simulink model "pointing_group24"  (R2023b)
settings: Solver=FixedStepAuto  StartTime=0.0  StopTime=T  RelTol=1e-3
values from neighbouring files (symbols this model uses):
  a = 6939    [Air_Drag_script.m]    (also in main.m = 6939.063; main_group24.m = 6978)
  AccMagn = 0.5    [main_group24.m]
  AccSunSens = 0.125    [main_group24.m]
  ARW = deg2rad(0.10)    [main_group24.m]
  by = 0.1    [main_group24.m]
  bz = 0.1    [main_group24.m]
  c = 2.99792*10^8    (= 299792000)    [main.m]    (also in main_group24.m = 299792458)
  Cd = 2.2    [main_group24.m]
  e = 0    [Air_Drag_script.m]    (also in main.m = 0.001304; main_group24.m)
  G = [gn, gm, gvali, gsvi]    [main.m]    (also in main_group24.m)
  GyroSampleRate = 10    [main_group24.m]
  H = [hn, hm, hvali, hsvi]    [main.m]    (also in main_group24.m)
  H_0 = ((g1_0^2)+(g1_1^2)+(h1_1^2))^0.5    (= 2.98059244128e-05)    [main_group24.m]
  i = deg2rad(97.5307)    [Air_Drag_script.m]    (also in main.m; main_group24.m = deg2rad(98))
  I_tot = [Ix 0 0; 0 Iy 0; 0 0 Iz]    [data_mass.m]    (also in main_group24.m)
  invI_tot = inv(I_tot)    [data_mass.m]    (also in main_group24.m)
  Ix = J(1,1)    [Air_Drag_script.m]    (also in data_mass.m = 0.0755003333333; main.m = 0.057749855; main_group24.m = 0.0755003333333)
  Iy = J(2,2)    [Air_Drag_script.m]    (also in data_mass.m = 0.0755003333333; main.m = 0.04143542; main_group24.m = 0.0755003333333)
  Iz = J(3,3)    [Air_Drag_script.m]    (also in data_mass.m = 0.055; main.m = 0.024624309; main_group24.m = 0.055)
  k1 = 5e-2    (= 0.05)    [main_group24.m]
  k2 = 2.5e-2    (= 0.025)    [main_group24.m]
  m = [0.1; 0.1; 0.1]    [main.m]    (also in main_group24.m)
  MB = [4; 0.1; 0.1; 0.3]    [main.m]    (also in main_group24.m)
  MMnoise = 15e-9*[1; 1; 1]    [main_group24.m]
  MMSampleRate = 1    [main_group24.m]
  mu = 3.98600433e+5    (= 398600.433)    [main.m]    (also in main_group24.m)
  n = 0.0011    [Air_Drag_script.m]    (also in main.m = sqrt(mu/a^3); main_group24.m = sqrt(mu/a^3))
  n_E = 729.2e-07    (= 7.292e-05)    [main_group24.m]
  om_E = 0.000072921    (= 7.2921e-05)    [main_group24.m]
  P = Fe/c    (= 4.52980041279e-06)    [main_group24.m]
  q0 = [ 1 1 1 1 ]'    [Air_Drag_script.m]    (also in main_group24.m = [0 0 0 1]')
  R_e = 6378    [main.m]    (also in main_group24.m)
  rho_air = 1.65e-13    [Air_Drag_script.m]    (also in main_group24.m = 6.967e-13)
  rho_d_body = 0.1*2/3    (= 0.0666666666667)    [main_group24.m]
  rho_d_sp = 0.1*2/3    (= 0.0666666666667)    [main_group24.m]
  rho_s_body = 0.5    [main_group24.m]
  rho_s_sp = 0.1    [main_group24.m]
  RRW = deg2rad(0.3)    [main_group24.m]
  SP = [1; 0.3; 0.1; 0.01]    [main.m]    (also in main_group24.m = [0.25; 0.1; 0.3; 0.01])
undefined symbols (not defined in the file or in its folder): pan, s1, s2, s3, s4, s5, s6, thrust
libraries: vrlib x25, matrix_library x17, simulink_extras x8, sharedutil x3, simulink x1
(part 2 of 5)

== system pointing_group24/Sensors1/Magnetometer/Subsystem ==
  Constant : Constant
  Display : Display
  Gain : Gain  Gain=[1; -1; 1]
  Gain1 : Gain  Gain=[1; 1; -1]
  Gain2 : Gain  Gain=[-1; 1; 1]
  Matrix Concatenate : Concatenate  NumInputs=3  Mode=Multidimensional array  ConcatenateDimension=2
  Random Number : RandomNumber  Variance=deg2rad(0.1)^2  Seed=5  SampleTime=1/MMSampleRate
  Random Number1 : RandomNumber  Variance=deg2rad(0.1)^2  Seed=6  SampleTime=1/MMSampleRate
  Random Number2 : RandomNumber  Variance=deg2rad(0.1)^2  Seed=7  SampleTime=1/MMSampleRate
  Selector : Selector  InputPortWidth=4  IndexOptions=Index vector (dialog)  Indices=[1 4 3]  OutputSizes=1
  Selector1 : Selector  InputPortWidth=4  IndexOptions=Index vector (dialog)  Indices=[4 1 2]  OutputSizes=1
  Selector2 : Selector  InputPortWidth=4  IndexOptions=Index vector (dialog)  Indices=[3 2 1]  OutputSizes=1
  Vector Concatenate : Concatenate  NumInputs=4
  A_epsMM : Outport
  wires:
  Selector2/1 -> Gain2/1
  Selector/1 -> Gain/1
  Gain/1 -> Matrix Concatenate/1
  Random Number/1 -> Vector Concatenate/2
  Matrix Concatenate/1 -> Display/1, A_epsMM/1
  Selector1/1 -> Gain1/1
  Vector Concatenate/1 -> Selector2/1, Selector/1, Selector1/1
  Gain2/1 -> Matrix Concatenate/3
  Constant/1 -> Vector Concatenate/1
  Gain1/1 -> Matrix Concatenate/2
  Random Number2/1 -> Vector Concatenate/4
  Random Number1/1 -> Vector Concatenate/3

== system pointing_group24/Sensors1/Sun Sensor/Subsystem ==
  note: A31
  note: A33
  note: A32
  note: A23
  note: A22
  note: A21
  note: A13
  note: A12
  note: A11
  Cos : Trigonometry  Operator=cos
  Cos1 : Trigonometry  Operator=cos
  Cos2 : Trigonometry  Operator=cos
  Create 3x3 Matrix : sharedutil/Create 3x3 Matrix  aMode=aMode
  Gain1 : Gain  Gain=-1
  Gain3 : Gain  Gain=-1
  Gain4 : Gain
  Product{,1,3,5..6,8,10..11} (8 alike) : Product
  Product{2,4,7,9} (4 alike) : Product  Inputs=3
  Sin : Trigonometry
  Sin1 : Trigonometry
  Sin2 : Trigonometry
  Sum : Sum
  Sum1 : Sum  Inputs=-+
  Sum2 : Sum  Inputs=-+
  Sum3 : Sum
  phi : RandomNumber  Variance=(1/8*pi/180)^2  Seed=2  SampleTime=0.2
  psi : RandomNumber  Variance=(1/8*pi/180)^2  SampleTime=0.2
  th : RandomNumber  Variance=(1/8*pi/180)^2  Seed=1  SampleTime=0.2
  A_eps : Outport
  wires:
  psi/1 -> Cos/1, Sin/1
  th/1 -> Sin1/1, Cos1/1
  phi/1 -> Sin2/1, Cos2/1
  Product2/1 -> Sum/1
  Product1/1 -> Sum/2
  Product3/1 -> Sum1/2
  Product4/1 -> Sum1/1
  Product7/1 -> Sum2/1
  Product6/1 -> Sum2/2
  Product9/1 -> Sum3/1
  Product8/1 -> Sum3/2
  Gain4/1 -> Create 3x3 Matrix/7  "A31"
  Product/1 -> Create 3x3 Matrix/1  "A11"
  Sum/1 -> Create 3x3 Matrix/2  "A12"
  Sum1/1 -> Create 3x3 Matrix/3  "A13"
  Product5/1 -> Gain1/1
  Sum2/1 -> Create 3x3 Matrix/5  "A22"
  Sum3/1 -> Create 3x3 Matrix/6  "A23"
  Product10/1 -> Gain3/1
  Product11/1 -> Create 3x3 Matrix/9  "A33"
  Gain1/1 -> Create 3x3 Matrix/4  "A21"
  Gain3/1 -> Create 3x3 Matrix/8  "A32"
  Cos/1 -> Product8/1, Product6/1, Product4/1, Product2/1, Product/1  "cos(psi)"
  Cos1/1 -> Product/2, Product11/1, Product10/1, Product5/2  "cos(th)"
  Sin1/1 -> Gain4/1, Product9/2, Product7/2, Product2/2, Product4/2  "sin(th)"
  Sin2/1 -> Product7/3, Product3/2, Product2/3, Product8/2, Product10/2  "sin(phi)"
  Sin/1 -> Product3/1, Product5/1, Product7/1, Product9/1, Product1/1  "sin(psi)"
  Cos2/1 -> Product6/2, Product4/3, Product1/2, Product9/3, Product11/2  "cos(phi)"
  Create 3x3 Matrix/1 -> A_eps/1  "A_eps"

== system pointing_group24/Attitude Control/Ideal controller/Subsystem2/Subsystem ==
  A11 : Inport
  A12 : Inport  Port=2
  A13 : Inport  Port=3
  A21 : Inport  Port=4
  A22 : Inport  Port=5
  A23 : Inport  Port=6
  A31 : Inport  Port=7
  A32 : Inport  Port=8
  A33 : Inport  Port=9
  Matrix Concatenate : Concatenate  NumInputs=3  Mode=Multidimensional array  ConcatenateDimension=2
  Mux : Mux  Inputs=3
  Mux1 : Mux  Inputs=3
  Mux2 : Mux  Inputs=3
  A_BN_312 : Outport
  wires:
  A31/1 -> Mux/3
  A13/1 -> Mux2/1
  Matrix Concatenate/1 -> A_BN_312/1
  Mux1/1 -> Matrix Concatenate/2
  A21/1 -> Mux/2
  A11/1 -> Mux/1
  A32/1 -> Mux1/3
  A12/1 -> Mux1/1
  Mux/1 -> Matrix Concatenate/1
  A33/1 -> Mux2/3
  A22/1 -> Mux1/2
  A23/1 -> Mux2/2
  Mux2/1 -> Matrix Concatenate/3

== system pointing_group24/Desturbances/External Torques/Air Drag/Subsystem ==
  v_rel_N^2 : Inport
  v_rel_B : Inport  Port=2
  Constant : Constant  Value=-0.5
  Constant1 : Constant  Value=s1.n
  Constant2 : Constant  Value=s1.r
  Constant3 : Constant  Value=s1.A
  Cross Product2 : vrlib/Utilities/Cross Product
  Dot Product1 : DotProduct  OutDataTypeStr=Inherit: Inherit via internal rule
  Gain : Gain  Gain=rho_air
  Gain1 : Gain  Gain=0
  Gain2 : Gain  Gain=Cd
  Product : Product  Inputs=5
  Switch1 : Switch  Criteria=u2 > Threshold  SaturateOnIntegerOverflow=off  InputSameDT=off
  Pan1 : Outport
  wires:
  Constant2/1 -> Cross Product2/1
  Gain1/1 -> Switch1/3
  Dot Product1/1 -> Gain1/1, Switch1/2, Switch1/1
  Constant3/1 -> Product/2
  Product/1 -> Cross Product2/2
  Switch1/1 -> Product/5
  v_rel_B/1 -> Dot Product1/1, Product/4
  Gain/1 -> Gain2/1
  Constant/1 -> Gain/1
  Cross Product2/1 -> Pan1/1
  Constant1/1 -> Dot Product1/2
  Gain2/1 -> Product/1
  v_rel_N^2/1 -> Product/3

== system pointing_group24/Desturbances/External Torques/Air Drag/Subsystem1 ==
  v_rel_N^2 : Inport
  v_rel_B : Inport  Port=2
  Constant : Constant  Value=-0.5
  Constant1 : Constant  Value=s2.n
  Constant2 : Constant  Value=s2.r
  Constant3 : Constant  Value=s2.A
  Cross Product2 : vrlib/Utilities/Cross Product
  Dot Product1 : DotProduct  OutDataTypeStr=Inherit: Inherit via internal rule
  Gain : Gain  Gain=rho_air
  Gain1 : Gain  Gain=0
  Gain2 : Gain  Gain=Cd
  Product : Product  Inputs=5
  Switch1 : Switch  Criteria=u2 > Threshold  SaturateOnIntegerOverflow=off  InputSameDT=off
  Pan2 : Outport
  wires:
  Constant1/1 -> Dot Product1/2
  Cross Product2/1 -> Pan2/1
  Constant/1 -> Gain/1
  Gain/1 -> Gain2/1
  Gain2/1 -> Product/1
  v_rel_B/1 -> Product/4, Dot Product1/1
  Switch1/1 -> Product/5
  Product/1 -> Cross Product2/2
  Constant3/1 -> Product/2
  Dot Product1/1 -> Switch1/1, Switch1/2, Gain1/1
  Gain1/1 -> Switch1/3
  Constant2/1 -> Cross Product2/1
  v_rel_N^2/1 -> Product/3

== system pointing_group24/Desturbances/External Torques/Air Drag/Subsystem2 ==
  v_rel_N^2 : Inport
  v_rel_B : Inport  Port=2
  Constant : Constant  Value=-0.5
  Constant1 : Constant  Value=s3.n
  Constant2 : Constant  Value=s3.r
  Constant3 : Constant  Value=s3.A
  Cross Product2 : vrlib/Utilities/Cross Product
  Dot Product1 : DotProduct  OutDataTypeStr=Inherit: Inherit via internal rule
  Gain : Gain  Gain=rho_air
  Gain1 : Gain  Gain=0
  Gain2 : Gain  Gain=Cd
  Product : Product  Inputs=5
  Switch1 : Switch  Criteria=u2 > Threshold  SaturateOnIntegerOverflow=off  InputSameDT=off
  Pan3 : Outport
  wires:
  Constant2/1 -> Cross Product2/1
  Gain1/1 -> Switch1/3
  Dot Product1/1 -> Gain1/1, Switch1/2, Switch1/1
  Constant3/1 -> Product/2
  Product/1 -> Cross Product2/2
  Switch1/1 -> Product/5
  v_rel_B/1 -> Dot Product1/1, Product/4
  Gain2/1 -> Product/1
  Gain/1 -> Gain2/1
  Constant/1 -> Gain/1
  Cross Product2/1 -> Pan3/1
  Constant1/1 -> Dot Product1/2
  v_rel_N^2/1 -> Product/3

== system pointing_group24/Desturbances/External Torques/Air Drag/Subsystem3 ==
  v_rel_N^2 : Inport
  v_rel_B : Inport  Port=2
  Constant : Constant  Value=-0.5
  Constant1 : Constant  Value=s4.n
  Constant2 : Constant  Value=s4.r
  Constant3 : Constant  Value=s4.A
  Cross Product2 : vrlib/Utilities/Cross Product
  Dot Product1 : DotProduct  OutDataTypeStr=Inherit: Inherit via internal rule
  Gain : Gain  Gain=rho_air
  Gain1 : Gain  Gain=0
  Gain2 : Gain  Gain=Cd
  Product : Product  Inputs=5
  Switch1 : Switch  Criteria=u2 > Threshold  SaturateOnIntegerOverflow=off  InputSameDT=off
  Pan4 : Outport
  wires:
  Constant1/1 -> Dot Product1/2
  Cross Product2/1 -> Pan4/1
  Constant/1 -> Gain/1
  Gain/1 -> Gain2/1
  Gain2/1 -> Product/1
  v_rel_B/1 -> Product/4, Dot Product1/1
  Switch1/1 -> Product/5
  Product/1 -> Cross Product2/2
  Constant3/1 -> Product/2
  Dot Product1/1 -> Switch1/1, Switch1/2, Gain1/1
  Gain1/1 -> Switch1/3
  Constant2/1 -> Cross Product2/1
  v_rel_N^2/1 -> Product/3

== system pointing_group24/Desturbances/External Torques/Air Drag/Subsystem4 ==
  v_rel_N^2 : Inport
  v_rel_B : Inport  Port=2
  Constant : Constant  Value=-0.5
  Constant1 : Constant  Value=s5.n
  Constant2 : Constant  Value=s5.r
  Constant3 : Constant  Value=s5.A
  Cross Product2 : vrlib/Utilities/Cross Product
  Dot Product1 : DotProduct  OutDataTypeStr=Inherit: Inherit via internal rule
  Gain : Gain  Gain=rho_air
  Gain1 : Gain  Gain=0
  Gain2 : Gain  Gain=Cd
  Product : Product  Inputs=5
  Switch1 : Switch  Criteria=u2 > Threshold  SaturateOnIntegerOverflow=off  InputSameDT=off
  Pan5 : Outport
  wires:
  Constant2/1 -> Cross Product2/1
  Gain1/1 -> Switch1/3
  Dot Product1/1 -> Gain1/1, Switch1/2, Switch1/1
  Constant3/1 -> Product/2
  Product/1 -> Cross Product2/2
  Switch1/1 -> Product/5
  v_rel_B/1 -> Dot Product1/1, Product/4
  Gain2/1 -> Product/1
  Gain/1 -> Gain2/1
  Constant/1 -> Gain/1
  Cross Product2/1 -> Pan5/1
  Constant1/1 -> Dot Product1/2
  v_rel_N^2/1 -> Product/3

== system pointing_group24/Desturbances/External Torques/Air Drag/Subsystem5 ==
  v_rel_N^2 : Inport
  v_rel_B : Inport  Port=2
  Constant : Constant  Value=-0.5
  Constant1 : Constant  Value=s6.n
  Constant2 : Constant  Value=s6.r
  Constant3 : Constant  Value=s6.A
  Cross Product2 : vrlib/Utilities/Cross Product
  Dot Product1 : DotProduct  OutDataTypeStr=Inherit: Inherit via internal rule
  Gain : Gain  Gain=rho_air
  Gain1 : Gain  Gain=0
  Gain2 : Gain  Gain=Cd
  Product : Product  Inputs=5
  Switch1 : Switch  Criteria=u2 > Threshold  SaturateOnIntegerOverflow=off  InputSameDT=off
  Pan6 : Outport
  wires:
  Constant2/1 -> Cross Product2/1
  Gain1/1 -> Switch1/3
  Dot Product1/1 -> Gain1/1, Switch1/2, Switch1/1
  Constant3/1 -> Product/2
  Product/1 -> Cross Product2/2
  Switch1/1 -> Product/5
  v_rel_B/1 -> Dot Product1/1, Product/4
  Gain2/1 -> Product/1
  Gain/1 -> Gain2/1
  Constant/1 -> Gain/1
  Cross Product2/1 -> Pan6/1
  Constant1/1 -> Dot Product1/2
  v_rel_N^2/1 -> Product/3

== system pointing_group24/Desturbances/External Torques/Air Drag/Subsystem6 ==
  v_rel_N^2 : Inport
  v_rel_B : Inport  Port=2
  Constant : Constant  Value=-0.5
  Constant1 : Constant  Value=pan.n1
  Constant2 : Constant  Value=pan.r
  Constant3 : Constant  Value=pan.A
  Cross Product2 : vrlib/Utilities/Cross Product
  Dot Product1 : DotProduct  OutDataTypeStr=Inherit: Inherit via internal rule
  Gain : Gain  Gain=rho_air
  Gain1 : Gain  Gain=0
  Gain2 : Gain  Gain=Cd
  Product : Product  Inputs=5
  Switch1 : Switch  Criteria=u2 > Threshold  SaturateOnIntegerOverflow=off  InputSameDT=off
  Ps1 : Outport
  wires:
  Constant1/1 -> Dot Product1/2
  Cross Product2/1 -> Ps1/1
  Constant/1 -> Gain/1
  Gain/1 -> Gain2/1
  Gain2/1 -> Product/1
  v_rel_B/1 -> Product/4, Dot Product1/1
  Switch1/1 -> Product/5
  Product/1 -> Cross Product2/2
  Constant3/1 -> Product/2
  Dot Product1/1 -> Switch1/1, Switch1/2, Gain1/1
  Gain1/1 -> Switch1/3
  Constant2/1 -> Cross Product2/1
  v_rel_N^2/1 -> Product/3

== system pointing_group24/Desturbances/External Torques/Air Drag/Subsystem7 ==
  v_rel_N^2 : Inport
  v_rel_B : Inport  Port=2
  Constant : Constant  Value=-0.5
  Constant1 : Constant  Value=pan.n2
  Constant2 : Constant  Value=pan.r
  Constant3 : Constant  Value=pan.A
  Cross Product2 : vrlib/Utilities/Cross Product
  Dot Product1 : DotProduct  OutDataTypeStr=Inherit: Inherit via internal rule
  Gain : Gain  Gain=rho_air
  Gain1 : Gain  Gain=0
  Gain2 : Gain  Gain=Cd
  Product : Product  Inputs=5
  Switch1 : Switch  Criteria=u2 > Threshold  SaturateOnIntegerOverflow=off  InputSameDT=off
  Ps2 : Outport
  wires:
  Constant2/1 -> Cross Product2/1
  Gain1/1 -> Switch1/3
  Dot Product1/1 -> Gain1/1, Switch1/2, Switch1/1
  Constant3/1 -> Product/2
  Product/1 -> Cross Product2/2
  Switch1/1 -> Product/5
  v_rel_B/1 -> Dot Product1/1, Product/4
  Gain2/1 -> Product/1
  Gain/1 -> Gain2/1
  Constant/1 -> Gain/1
  Cross Product2/1 -> Ps2/1
  Constant1/1 -> Dot Product1/2
  v_rel_N^2/1 -> Product/3

== system pointing_group24/Desturbances/External Torques/M_GG/GG Torque1 ==
  c1 : Inport
  c2 : Inport  Port=2
  c3 : Inport  Port=3
  r : Inport  Port=4
  Constant5 : Constant  Value=3
  Constant6 : Constant  Value=3*mu
  Divide3 : Product  Inputs=*/
  Gain1 : Gain  Gain=Iz-Iy
  Gain2 : Gain  Gain=Ix-Iz
  Gain3 : Gain  Gain=Iy-Ix
  Mux1 : Mux  Inputs=3
  Pow1 : Math  Operator=pow  RndMeth=Zero
  Product{1..2,6..9} (6 alike) : Product
  M_GG : Outport
  wires:
  Gain1/1 -> Mux1/1
  Product7/1 -> Gain1/1
  Gain3/1 -> Mux1/3
  Product2/1 -> Product8/1
  r/1 -> Pow1/1
  Product6/1 -> Product9/1
  Product1/1 -> Product7/1
  Constant6/1 -> Divide3/1
  Product8/1 -> Gain2/1
  Pow1/1 -> Divide3/2
  c2/1 -> Product6/2, Product1/1
  Mux1/1 -> M_GG/1
  Product9/1 -> Gain3/1
  Constant5/1 -> Pow1/2
  Gain2/1 -> Mux1/2
  c3/1 -> Product1/2, Product2/2
  c1/1 -> Product6/1, Product2/1
  Divide3/1 -> Product7/2, Product8/2, Product9/2

== system pointing_group24/Desturbances/External Torques/M_GG/c1, c2, c3 ==
  A_BL : Inport
  Constant1 : Constant  Value=[1; 0; 0]
  Demux : Demux  Outputs=3
  Product1 : Product  Multiplication=Matrix(*)
  c1 : Outport
  c2 : Outport  Port=2
  c3 : Outport  Port=3
  wires:
  Demux/2 -> c2/1
  Product1/1 -> Demux/1
  Demux/1 -> c1/1
  Demux/3 -> c3/1
  Constant1/1 -> Product1/2
  A_BL/1 -> Product1/1

== system pointing_group24/Desturbances/External Torques/Reflected radiation/Areas ==
  MB : Inport
  Demux : Demux
  Mux : Mux  Inputs=3
  Product1 : Product
  Product2 : Product
  Product4 : Product
  Reshape : Reshape  OutputDimensionality=Column vector (2-D)
  Terminator : Terminator
  A_vect : Outport
  wires:
  Reshape/1 -> A_vect/1
  Mux/1 -> Reshape/1
  [a] -> Product1/1
  [a] -> Product2/1
  [b] -> Product1/2
  [h] -> Product2/2
  [h] -> Product4/2
  [b] -> Product4/1
  Demux/4 -> [h]
  Demux/3 -> [b]
  Demux/2 -> [a]
  Demux/1 -> Terminator/1
  Product1/1 -> Mux/3  "a*b"
  MB/1 -> Demux/1
  Product4/1 -> Mux/1  "b*h"
  Product2/1 -> Mux/2  "a*h"

== system pointing_group24/Desturbances/External Torques/Reflected radiation/Areas_SP ==
  SP : Inport
  Demux : Demux
  Product1 : Product
  Terminator : Terminator
  Terminator1 : Terminator
  A_vect : Outport
  wires:
  SP/1 -> Demux/1
  Product1/1 -> A_vect/1  "a*b"
  Demux/1 -> Terminator/1
  Demux/2 -> [a]
  Demux/3 -> [b]
  Demux/4 -> Terminator1/1
  [b] -> Product1/2
  [a] -> Product1/1

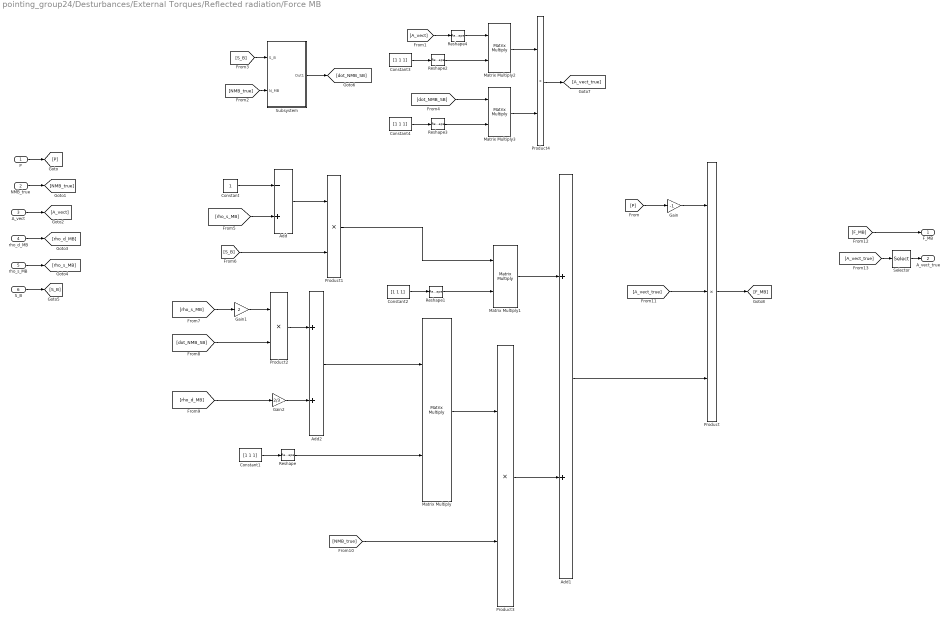
== system pointing_group24/Desturbances/External Torques/Reflected radiation/Force MB ==
  P : Inport
  NMB_true : Inport  Port=2
  A_vect : Inport  Port=3
  rho_d_MB : Inport  Port=4
  rho_s_MB : Inport  Port=5
  S_B : Inport  Port=6
  Add : Sum  Inputs=-+
  Add1 : Sum
  Add2 : Sum
  Constant : Constant
  Constant{1..4} (4 alike) : Constant  Value=[1 1 1]
  Gain : Gain  Gain=-1
  Gain1 : Gain  Gain=2
  Gain2 : Gain  Gain=2/3
  Matrix Multiply{,1..3} (4 alike) : Product  Multiplication=Matrix(*)
  Product : Product  Inputs=3
  Product{1..4} (4 alike) : Product
  Reshape{,1..3} (4 alike) : Reshape  OutputDimensionality=Row vector (2-D)
  Reshape4 : Reshape  OutputDimensionality=Column vector (2-D)
  Selector : Selector  NumberOfDimensions=2  InputPortWidth=3  IndexOptions=Index vector (dialog),Index vector (dialog)  Indices=[1 2 3],1  OutputSizes=1,1
  Subsystem : Subsystem
  F_MB : Outport
  A_vect_true : Outport  Port=2
  wires:
  Selector/1 -> A_vect_true/1
  [A_vect_true] -> Selector/1
  [F_MB] -> F_MB/1
  Product/1 -> [F_MB]
  [A_vect_true] -> Product/2
  Product4/1 -> [A_vect_true]
  Matrix Multiply3/1 -> Product4/2
  Matrix Multiply2/1 -> Product4/1
  [dot_NMB_SB] -> Matrix Multiply3/1
  Reshape4/1 -> Matrix Multiply2/1
  [A_vect] -> Reshape4/1
  Constant4/1 -> Reshape3/1
  Reshape3/1 -> Matrix Multiply3/2
  Constant3/1 -> Reshape2/1
  Reshape2/1 -> Matrix Multiply2/2
  Reshape1/1 -> Matrix Multiply1/2
  Constant2/1 -> Reshape1/1
  Product1/1 -> Matrix Multiply1/1
  Matrix Multiply1/1 -> Add1/1
  Reshape/1 -> Matrix Multiply/2
  Add2/1 -> Matrix Multiply/1
  Matrix Multiply/1 -> Product3/1
  Constant1/1 -> Reshape/1
  Add1/1 -> Product/3
  Product3/1 -> Add1/2
  [NMB_true] -> Product3/2
  [rho_d_MB] -> Gain2/1
  Gain2/1 -> Add2/2
  Product2/1 -> Add2/1
  Gain1/1 -> Product2/1
  [dot_NMB_SB] -> Product2/2
  [rho_s_MB] -> Gain1/1
  [S_B] -> Product1/2
  Add/1 -> Product1/1
  Constant/1 -> Add/1
  [rho_s_MB] -> Add/2
  Subsystem/1(Out1) -> [dot_NMB_SB]
  [S_B] -> Subsystem/1(S_B)
  [NMB_true] -> Subsystem/2(N_MB)
  Gain/1 -> Product/1
  [P] -> Gain/1
  S_B/1 -> [S_B]
  rho_s_MB/1 -> [rho_s_MB]
  rho_d_MB/1 -> [rho_d_MB]
  A_vect/1 -> [A_vect]
  NMB_true/1 -> [NMB_true]
  P/1 -> [P]

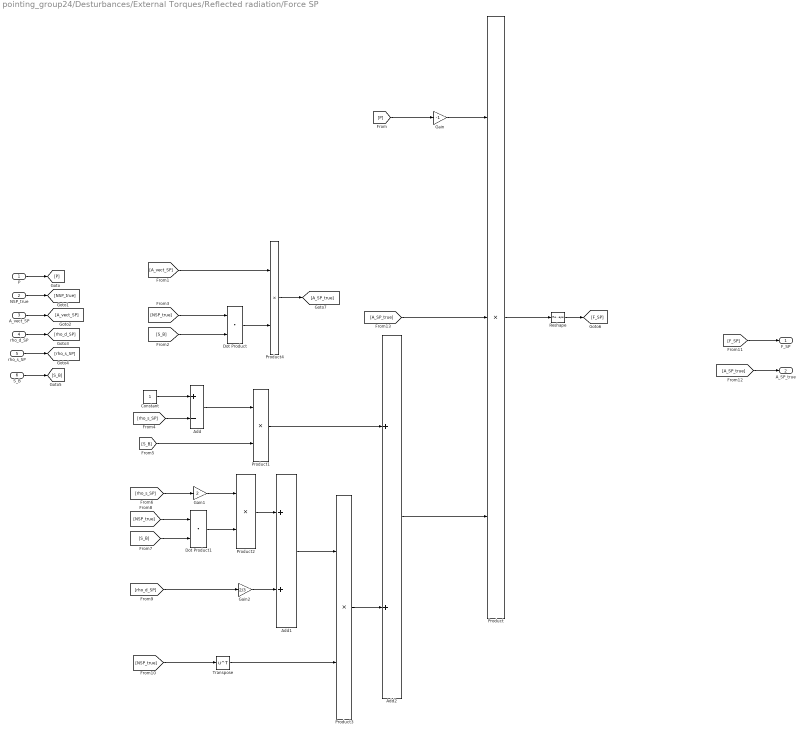
== system pointing_group24/Desturbances/External Torques/Reflected radiation/Force SP ==
  P : Inport
  NSP_true : Inport  Port=2
  A_vect_SP : Inport  Port=3
  rho_d_SP : Inport  Port=4
  rho_s_SP : Inport  Port=5
  S_B : Inport  Port=6
  Add : Sum  Inputs=+-
  Add1 : Sum
  Add2 : Sum
  Constant : Constant
  Dot Product : DotProduct  OutDataTypeStr=Inherit: Inherit via internal rule
  Dot Product1 : DotProduct  OutDataTypeStr=Inherit: Inherit via internal rule
  Gain : Gain  Gain=-1
  Gain1 : Gain  Gain=2
  Gain2 : Gain  Gain=2/3
  Product : Product  Inputs=3
  Product{1..4} (4 alike) : Product
  Reshape : Reshape  OutputDimensionality=Row vector (2-D)
  Transpose : Math  Operator=transpose
  F_SP : Outport
  A_SP_true : Outport  Port=2
  wires:
  [A_SP_true] -> Product/2
  [A_SP_true] -> A_SP_true/1
  Product4/1 -> [A_SP_true]
  [A_vect_SP] -> Product4/1
  Dot Product/1 -> Product4/2
  [F_SP] -> F_SP/1
  Reshape/1 -> [F_SP]
  Add2/1 -> Product/3
  Transpose/1 -> Product3/2
  Product3/1 -> Add2/2
  Product1/1 -> Add2/1
  Add1/1 -> Product3/1
  [NSP_true] -> Transpose/1
  Gain2/1 -> Add1/2
  [rho_d_SP] -> Gain2/1
  Product2/1 -> Add1/1
  Gain1/1 -> Product2/1
  Dot Product1/1 -> Product2/2
  [S_B] -> Dot Product1/2
  [NSP_true] -> Dot Product1/1
  [rho_s_SP] -> Gain1/1
  [S_B] -> Product1/2
  Add/1 -> Product1/1
  [rho_s_SP] -> Add/2
  Constant/1 -> Add/1
  [NSP_true] -> Dot Product/1
  [S_B] -> Dot Product/2
  Gain/1 -> Product/1
  [P] -> Gain/1
  Product/1 -> Reshape/1
  S_B/1 -> [S_B]
  rho_s_SP/1 -> [rho_s_SP]
  rho_d_SP/1 -> [rho_d_SP]
  A_vect_SP/1 -> [A_vect_SP]
  NSP_true/1 -> [NSP_true]
  P/1 -> [P]

== system pointing_group24/Desturbances/External Torques/Reflected radiation/Pressure ==
  Constant6 : Constant  Value=723
  Constant7 : Constant  Value=c
  Product8 : Product
  Reciprocal : Product  Inputs=/
  P : Outport
  wires:
  Constant7/1 -> Reciprocal/1
  Product8/1 -> P/1
  Reciprocal/1 -> Product8/2
  Constant6/1 -> Product8/1

== system pointing_group24/Desturbances/External Torques/Reflected radiation/SP center arm ==
  MB : Inport
  SP : Inport  Port=2
  Demux : Demux
  Demux1 : Demux
  Terminator{1..5} (5 alike) : Terminator
  r_SPx : Subsystem
  r_SPy : Subsystem
  r_SP1 : Outport
  r_SP2 : Outport  Port=2
  r_SP3 : Outport  Port=3
  r_SP4 : Outport  Port=4
  wires:
  [b_MB] -> r_SPy/2(b_MB)
  r_SPy/2(r_SP2) -> r_SP4/1
  [b_SP] -> r_SPy/1(b_SP)
  r_SPy/1(r_SP1) -> r_SP3/1
  r_SPx/1(r_SP1) -> r_SP1/1
  [b_SP] -> r_SPx/1(b_SP)
  Demux/3 -> [b_SP]
  r_SPx/2(r_SP2) -> r_SP2/1
  Demux/2 -> Terminator4/1
  Demux/4 -> Terminator3/1
  MB/1 -> Demux1/1
  Demux1/4 -> Terminator1/1
  Demux1/1 -> Terminator2/1
  Demux1/3 -> [b_MB]
  Demux1/2 -> [a_MB]
  SP/1 -> Demux/1
  Demux/1 -> Terminator5/1
  [a_MB] -> r_SPx/2(a_MB)

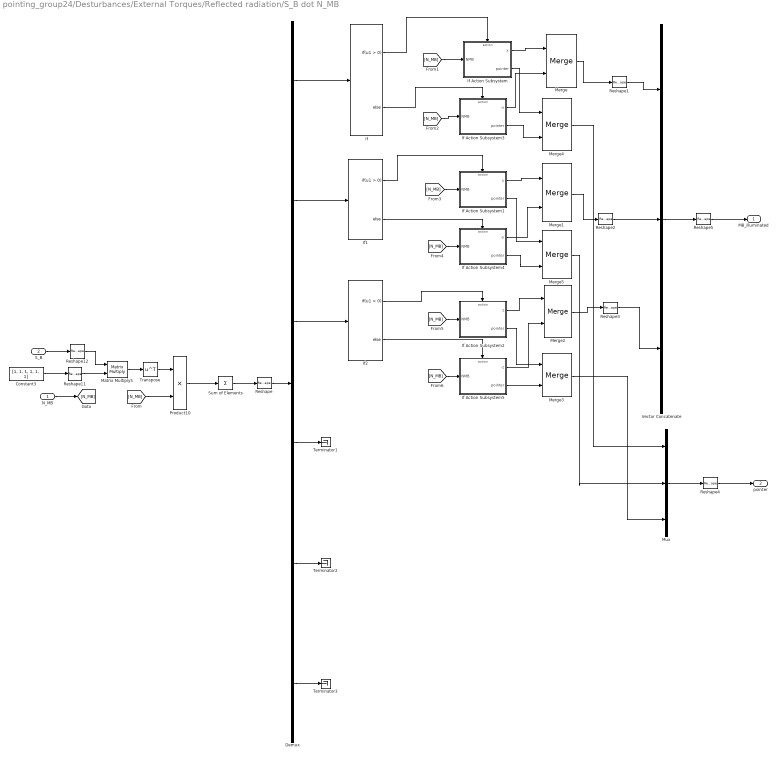
== system pointing_group24/Desturbances/External Torques/Reflected radiation/S_B dot N_MB ==
  N_MB : Inport
  S_B : Inport  Port=2
  Constant3 : Constant  Value=[1, 1, 1, 1, 1, 1]  VectorParams1D=off
  Demux : Demux  Outputs=6
  If : If
  If Action Subsystem : Subsystem  TreatAsAtomicUnit=on
  If Action Subsystem1 : Subsystem  TreatAsAtomicUnit=on
  If Action Subsystem2 : Subsystem  TreatAsAtomicUnit=on
  If Action Subsystem3 : Subsystem  TreatAsAtomicUnit=on
  If Action Subsystem4 : Subsystem  TreatAsAtomicUnit=on
  If Action Subsystem5 : Subsystem  TreatAsAtomicUnit=on
  If1 : If
  If2 : If
  Matrix Multiply5 : Product  Multiplication=Matrix(*)
  Merge{,1..5} (6 alike) : Merge
  Mux : Mux  Inputs=3
  Product10 : Product
  Reshape{,1..4,12} (6 alike) : Reshape  OutputDimensionality=Column vector (2-D)
  Reshape11 : Reshape  OutputDimensionality=Row vector (2-D)
  Reshape5 : Reshape  OutputDimensionality=Customize  OutputDimensions=[3,3]
  Sum of Elements : Sum  Inputs=+  CollapseMode=Specified dimension  CollapseDim=2
  Terminator1 : Terminator
  Terminator2 : Terminator
  Terminator3 : Terminator
  Transpose : Math  Operator=transpose
  Vector Concatenate : Concatenate  NumInputs=3
  MB_illuminated : Outport
  pointer : Outport  Port=2
  wires:
  Transpose/1 -> Product10/1
  Reshape5/1 -> MB_illuminated/1
  Reshape4/1 -> pointer/1
  Mux/1 -> Reshape4/1
  Merge3/1 -> Mux/3
  Merge5/1 -> Mux/2
  Merge4/1 -> Mux/1
  If Action Subsystem5/2(pointer) -> Merge3/2
  If Action Subsystem2/2(pointer) -> Merge3/1
  If Action Subsystem4/2(pointer) -> Merge5/2
  If Action Subsystem1/2(pointer) -> Merge5/1
  If Action Subsystem3/2(pointer) -> Merge4/2
  If Action Subsystem/2(pointer) -> Merge4/1
  If Action Subsystem4/1(-y) -> Merge1/2
  Vector Concatenate/1 -> Reshape5/1
  Reshape3/1 -> Vector Concatenate/3
  Reshape2/1 -> Vector Concatenate/2
  Reshape1/1 -> Vector Concatenate/1
  Merge2/1 -> Reshape3/1
  Merge1/1 -> Reshape2/1
  Merge/1 -> Reshape1/1
  [N_MB] -> If Action Subsystem5/1(NMB)
  [N_MB] -> If Action Subsystem2/1(NMB)
  If2/2 -> If Action Subsystem5/Action
  If2/1 -> If Action Subsystem2/Action
  Demux/3 -> If2/1
  If Action Subsystem5/1(-z) -> Merge2/2
  If Action Subsystem2/1(z) -> Merge2/1
  If Action Subsystem1/1(y) -> Merge1/1
  If Action Subsystem/1(x) -> Merge/1
  If Action Subsystem3/1(-x) -> Merge/2
  [N_MB] -> If Action Subsystem4/1(NMB)
  If1/2 -> If Action Subsystem4/Action
  [N_MB] -> If Action Subsystem1/1(NMB)
  [N_MB] -> If Action Subsystem3/1(NMB)
  If1/1 -> If Action Subsystem1/Action
  Demux/2 -> If1/1
  Demux/6 -> Terminator3/1
  Demux/5 -> Terminator2/1
  Demux/4 -> Terminator1/1
  [N_MB] -> If Action Subsystem/1(NMB)
  [N_MB] -> Product10/2
  N_MB/1 -> [N_MB]
  If/2 -> If Action Subsystem3/Action
  If/1 -> If Action Subsystem/Action
  Demux/1 -> If/1
  Reshape/1 -> Demux/1
  Sum of Elements/1 -> Reshape/1
  S_B/1 -> Reshape12/1
  Constant3/1 -> Reshape11/1
  Reshape11/1 -> Matrix Multiply5/2
  Product10/1 -> Sum of Elements/1
  Matrix Multiply5/1 -> Transpose/1
  Reshape12/1 -> Matrix Multiply5/1

== system pointing_group24/Desturbances/External Torques/Reflected radiation/S_B dot N_SP ==
  N_SP : Inport
  S_B : Inport  Port=2
  Constant3 : Constant  Value=[1, 1, 1, 1]
  Demux : Demux
  If : If
  If Action Subsystem : Subsystem  TreatAsAtomicUnit=on
  If Action Subsystem1 : Subsystem  TreatAsAtomicUnit=on
  If1 : If
  Matrix Multiply5 : Product  Multiplication=Matrix(*)
  Merge : Merge
  Merge1 : Merge
  Product10 : Product
  Reshape11 : Reshape  OutputDimensionality=Row vector (2-D)
  Reshape12 : Reshape  OutputDimensionality=Column vector (2-D)
  Sum of Elements : Sum  Inputs=+  CollapseMode=Specified dimension  CollapseDim=2
  Terminator{,1..3} (4 alike) : Terminator
  Transpose : Math  Operator=transpose
  SP_illuminated : Outport
  pointer : Outport  Port=2
  wires:
  Demux/4 -> Terminator3/1
  Demux/3 -> Terminator2/1
  Merge1/1 -> pointer/1
  Merge/1 -> SP_illuminated/1
  If Action Subsystem1/2(pointer) -> Merge1/2
  If Action Subsystem/2(pointer) -> Merge1/1
  If Action Subsystem1/1(true_NSP) -> Merge/2
  If Action Subsystem/1(true_NSP) -> Merge/1
  If/2 -> Terminator1/1
  If1/2 -> Terminator/1
  If1/1 -> If Action Subsystem1/Action
  [N_SP] -> If Action Subsystem1/1(N_SP)
  [N_SP] -> If Action Subsystem/1(N_SP)
  Demux/2 -> If1/1
  If/1 -> If Action Subsystem/Action
  Demux/1 -> If/1
  Transpose/1 -> Product10/1
  Reshape12/1 -> Matrix Multiply5/1
  Matrix Multiply5/1 -> Transpose/1
  Product10/1 -> Sum of Elements/1
  Reshape11/1 -> Matrix Multiply5/2
  Constant3/1 -> Reshape11/1
  S_B/1 -> Reshape12/1
  Sum of Elements/1 -> Demux/1
  N_SP/1 -> [N_SP]
  [N_SP] -> Product10/2

== system pointing_group24/Desturbances/External Torques/Reflected radiation/Torque arm MB ==
  note: creo il vettore somma che ha per colonna i raggi vettori che collegano il CM del MB con i centri illuminati delle facce nel caso che il sole sia nelle 4 posizioni.
  MB : Inport
  A_vect : Inport  Port=2
  S_B : Inport  Port=3
  pointer : Inport  Port=4
  Demux : Demux  Outputs=3
  Reshape : Reshape  OutputDimensionality=Customize  OutputDimensions=[3,3]
  Transpose : Math  Operator=transpose
  Vector Concatenate : Concatenate  NumInputs=3
  creazione raggi vettore tra CM MB e centro facce illuminate della faccia che ha come normale l'asse i : Subsystem
  creazione raggi vettore tra CM MB e centro facce illuminate della faccia che ha come normale l'asse j : Subsystem
  creazione raggi vettore tra CM MB e centro facce illuminate della faccia che ha come normale l'asse k : Subsystem
  dist : Outport
  wires:
  creazione raggi vettore tra CM MB e centro facce illuminate della faccia che ha come normale l'asse i/1(Out1) -> Vector Concatenate/1
  creazione raggi vettore tra CM MB e centro facce illuminate della faccia che ha come normale l'asse j/1(Out1) -> Vector Concatenate/2
  creazione raggi vettore tra CM MB e centro facce illuminate della faccia che ha come normale l'asse k/1(Out1) -> Vector Concatenate/3
  Demux/2 -> [y]
  [S_B] -> creazione raggi vettore tra CM MB e centro facce illuminate della faccia che ha come normale l'asse i/1(S_B)
  [A_vect] -> creazione raggi vettore tra CM MB e centro facce illuminate della faccia che ha come normale l'asse j/3(A_vect)
  Vector Concatenate/1 -> Reshape/1  "vectors x, y, z"
  [z] -> creazione raggi vettore tra CM MB e centro facce illuminate della faccia che ha come normale l'asse k/4(pointer)
  [S_B] -> creazione raggi vettore tra CM MB e centro facce illuminate della faccia che ha come normale l'asse j/1(S_B)
  Demux/3 -> [z]
  Demux/1 -> [x]
  [S_B] -> creazione raggi vettore tra CM MB e centro facce illuminate della faccia che ha come normale l'asse k/1(S_B)
  Transpose/1 -> dist/1
  Reshape/1 -> Transpose/1
  [MB] -> creazione raggi vettore tra CM MB e centro facce illuminate della faccia che ha come normale l'asse i/2(MB)
  MB/1 -> [MB]
  A_vect/1 -> [A_vect]
  [MB] -> creazione raggi vettore tra CM MB e centro facce illuminate della faccia che ha come normale l'asse j/2(MB)
  [A_vect] -> creazione raggi vettore tra CM MB e centro facce illuminate della faccia che ha come normale l'asse k/3(A_vect)
  S_B/1 -> [S_B]
  [y] -> creazione raggi vettore tra CM MB e centro facce illuminate della faccia che ha come normale l'asse j/4(pointer)
  [MB] -> creazione raggi vettore tra CM MB e centro facce illuminate della faccia che ha come normale l'asse k/2(MB)
  [A_vect] -> creazione raggi vettore tra CM MB e centro facce illuminate della faccia che ha come normale l'asse i/3(A_vect)
  [x] -> creazione raggi vettore tra CM MB e centro facce illuminate della faccia che ha come normale l'asse i/4(pointer)
  pointer/1 -> Demux/1

== system pointing_group24/Desturbances/External Torques/Reflected radiation/Torque arm SP ==
  SP : Inport
  A_vect_SP : Inport  Port=2
  S_B : Inport  Port=3
  pointer_SP : Inport  Port=4
  r_SP1 : Inport  Port=5
  r_SP2 : Inport  Port=6
  r_SP3 : Inport  Port=7
  r_SP4 : Inport  Port=8
  Add{,1..3} (4 alike) : Sum
  Reshape : Reshape  OutputDimensionality=Customize  OutputDimensions=[4,3]
  Vector Concatenate : Concatenate  NumInputs=4
  creazione raggi vettore tra CM SP e centro di pressione della faccia illuminata : Subsystem
  distance : Outport
  wires:
  creazione raggi vettore tra CM SP e centro di pressione della faccia illuminata/2(distance_y) -> [distance_y]
  Add3/1 -> Vector Concatenate/4
  [distance_y] -> Add3/1
  [r_SP4] -> Add3/2
  [r_SP3] -> Add2/2
  [distance_y] -> Add2/1
  Add2/1 -> Vector Concatenate/3
  r_SP4/1 -> [r_SP4]
  r_SP3/1 -> [r_SP3]
  Add1/1 -> Vector Concatenate/2
  [distance_x] -> Add1/1
  [r_SP2] -> Add1/2
  [r_SP1] -> Add/2
  [distance_x] -> Add/1
  Add/1 -> Vector Concatenate/1
  Vector Concatenate/1 -> Reshape/1
  creazione raggi vettore tra CM SP e centro di pressione della faccia illuminata/1(distance_x) -> [distance_x]
  [pointer_SP] -> creazione raggi vettore tra CM SP e centro di pressione della faccia illuminata/4(pointer)
  [A_vect_SP] -> creazione raggi vettore tra CM SP e centro di pressione della faccia illuminata/3(A_vect)
  [SP] -> creazione raggi vettore tra CM SP e centro di pressione della faccia illuminata/2(SP)
  [S_B] -> creazione raggi vettore tra CM SP e centro di pressione della faccia illuminata/1(S_B)
  r_SP2/1 -> [r_SP2]
  r_SP1/1 -> [r_SP1]
  pointer_SP/1 -> [pointer_SP]
  S_B/1 -> [S_B]
  A_vect_SP/1 -> [A_vect_SP]
  SP/1 -> [SP]
  Reshape/1 -> distance/1

== system pointing_group24/Desturbances/External Torques/SRP con frecce/SRP ==
  S_B : Inport
  Gain : Gain  Gain=4
  Gain1 : Gain  Gain=4
  Subsystem : Subsystem
  Subsystem1 : Subsystem
  Subsystem2 : Subsystem
  Subsystem3 : Subsystem
  Subsystem4 : Subsystem
  Subsystem5 : Subsystem
  Subsystem6 : Subsystem
  Subsystem7 : Subsystem
  Sum : Sum  Inputs=++++++++
  Tsrp : Outport
  wires:
  S_B/1 -> Subsystem2/1(S_B), Subsystem/1(S_B), Subsystem1/1(S_B), Subsystem4/1(S_B), Subsystem3/1(S_B), Subsystem7/1(S_B), Subsystem5/1(S_B), Subsystem6/1(S_B)
  Subsystem2/1(pan1) -> Sum/1
  Subsystem/1(pan2) -> Sum/2
  Subsystem1/1(pan3) -> Sum/3
  Subsystem4/1(pan4) -> Sum/4
  Subsystem3/1(pan5) -> Sum/5
  Subsystem7/1(pan6) -> Sum/6
  Sum/1 -> Tsrp/1
  Subsystem5/1(ps1) -> Gain/1
  Gain/1 -> Sum/7
  Subsystem6/1(ps2) -> Gain1/1
  Gain1/1 -> Sum/8

== system pointing_group24/Desturbances/External Torques/Solar radiation/Areas ==
  MB : Inport
  Demux : Demux
  Mux : Mux  Inputs=3
  Product1 : Product
  Product2 : Product
  Product4 : Product
  Reshape : Reshape  OutputDimensionality=Column vector (2-D)
  Terminator : Terminator
  A_vect : Outport
  wires:
  Product2/1 -> Mux/2  "a*h"
  Product4/1 -> Mux/1  "b*h"
  MB/1 -> Demux/1
  Product1/1 -> Mux/3  "a*b"
  Demux/1 -> Terminator/1
  Demux/2 -> [a]
  Demux/3 -> [b]
  Demux/4 -> [h]
  [b] -> Product4/1
  [h] -> Product4/2
  [h] -> Product2/2
  [b] -> Product1/2
  [a] -> Product2/1
  [a] -> Product1/1
  Mux/1 -> Reshape/1
  Reshape/1 -> A_vect/1

== system pointing_group24/Desturbances/External Torques/Solar radiation/Areas_SP ==
  SP : Inport
  Demux : Demux
  Product1 : Product
  Terminator : Terminator
  Terminator1 : Terminator
  A_vect : Outport
  wires:
  [a] -> Product1/1
  [b] -> Product1/2
  Demux/4 -> Terminator1/1
  Demux/3 -> [b]
  Demux/2 -> [a]
  Demux/1 -> Terminator/1
  Product1/1 -> A_vect/1  "a*b"
  SP/1 -> Demux/1

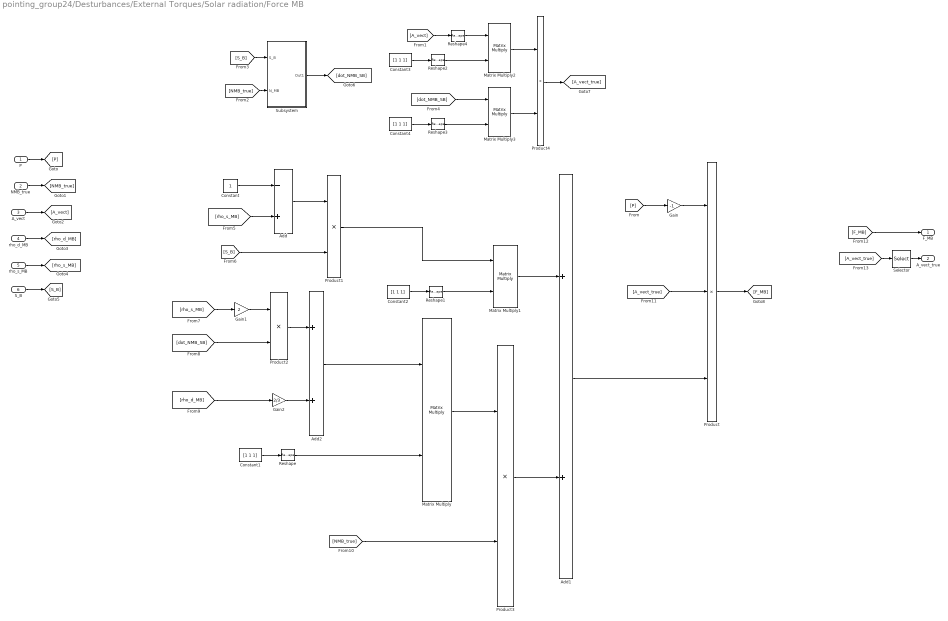
== system pointing_group24/Desturbances/External Torques/Solar radiation/Force MB ==
  P : Inport
  NMB_true : Inport  Port=2
  A_vect : Inport  Port=3
  rho_d_MB : Inport  Port=4
  rho_s_MB : Inport  Port=5
  S_B : Inport  Port=6
  Add : Sum  Inputs=-+
  Add1 : Sum
  Add2 : Sum
  Constant : Constant
  Constant{1..4} (4 alike) : Constant  Value=[1 1 1]
  Gain : Gain  Gain=-1
  Gain1 : Gain  Gain=2
  Gain2 : Gain  Gain=2/3
  Matrix Multiply{,1..3} (4 alike) : Product  Multiplication=Matrix(*)
  Product : Product  Inputs=3
  Product{1..4} (4 alike) : Product
  Reshape{,1..3} (4 alike) : Reshape  OutputDimensionality=Row vector (2-D)
  Reshape4 : Reshape  OutputDimensionality=Column vector (2-D)
  Selector : Selector  NumberOfDimensions=2  InputPortWidth=3  IndexOptions=Index vector (dialog),Index vector (dialog)  Indices=[1 2 3],1  OutputSizes=1,1
  Subsystem : Subsystem
  F_MB : Outport
  A_vect_true : Outport  Port=2
  wires:
  P/1 -> [P]
  NMB_true/1 -> [NMB_true]
  A_vect/1 -> [A_vect]
  rho_d_MB/1 -> [rho_d_MB]
  rho_s_MB/1 -> [rho_s_MB]
  S_B/1 -> [S_B]
  [P] -> Gain/1
  Gain/1 -> Product/1
  [NMB_true] -> Subsystem/2(N_MB)
  [S_B] -> Subsystem/1(S_B)
  Subsystem/1(Out1) -> [dot_NMB_SB]
  [rho_s_MB] -> Add/2
  Constant/1 -> Add/1
  Add/1 -> Product1/1
  [S_B] -> Product1/2
  [rho_s_MB] -> Gain1/1
  [dot_NMB_SB] -> Product2/2
  Gain1/1 -> Product2/1
  Product2/1 -> Add2/1
  Gain2/1 -> Add2/2
  [rho_d_MB] -> Gain2/1
  [NMB_true] -> Product3/2
  Product3/1 -> Add1/2
  Add1/1 -> Product/3
  Constant1/1 -> Reshape/1
  Matrix Multiply/1 -> Product3/1
  Add2/1 -> Matrix Multiply/1
  Reshape/1 -> Matrix Multiply/2
  Matrix Multiply1/1 -> Add1/1
  Product1/1 -> Matrix Multiply1/1
  Constant2/1 -> Reshape1/1
  Reshape1/1 -> Matrix Multiply1/2
  Reshape2/1 -> Matrix Multiply2/2
  Constant3/1 -> Reshape2/1
  Reshape3/1 -> Matrix Multiply3/2
  Constant4/1 -> Reshape3/1
  [A_vect] -> Reshape4/1
  Reshape4/1 -> Matrix Multiply2/1
  [dot_NMB_SB] -> Matrix Multiply3/1
  Matrix Multiply2/1 -> Product4/1
  Matrix Multiply3/1 -> Product4/2
  Product4/1 -> [A_vect_true]
  [A_vect_true] -> Product/2
  Product/1 -> [F_MB]
  [F_MB] -> F_MB/1
  [A_vect_true] -> Selector/1
  Selector/1 -> A_vect_true/1

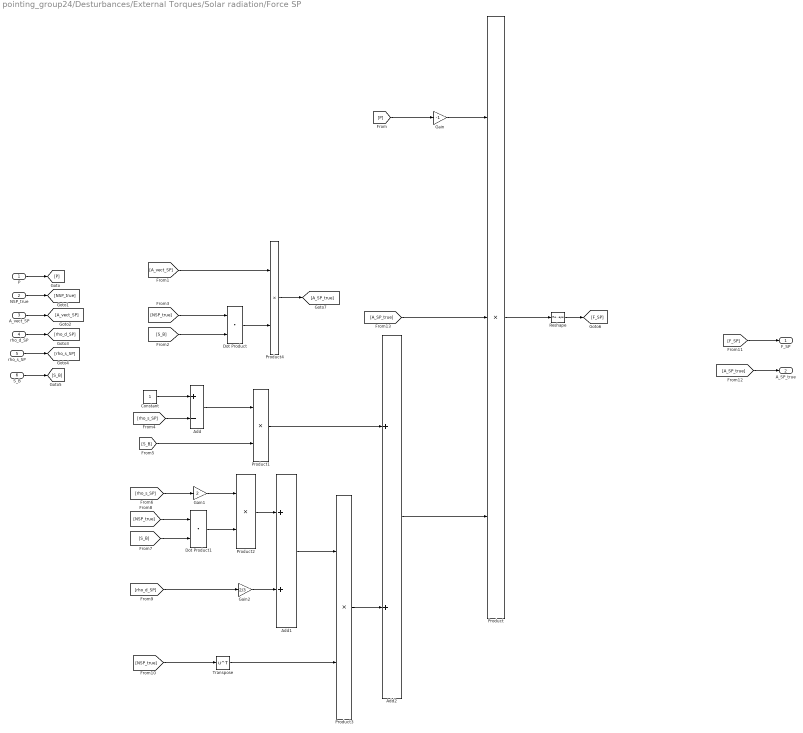
== system pointing_group24/Desturbances/External Torques/Solar radiation/Force SP ==
  P : Inport
  NSP_true : Inport  Port=2
  A_vect_SP : Inport  Port=3
  rho_d_SP : Inport  Port=4
  rho_s_SP : Inport  Port=5
  S_B : Inport  Port=6
  Add : Sum  Inputs=+-
  Add1 : Sum
  Add2 : Sum
  Constant : Constant
  Dot Product : DotProduct  OutDataTypeStr=Inherit: Inherit via internal rule
  Dot Product1 : DotProduct  OutDataTypeStr=Inherit: Inherit via internal rule
  Gain : Gain  Gain=-1
  Gain1 : Gain  Gain=2
  Gain2 : Gain  Gain=2/3
  Product : Product  Inputs=3
  Product{1..4} (4 alike) : Product
  Reshape : Reshape  OutputDimensionality=Row vector (2-D)
  Transpose : Math  Operator=transpose
  F_SP : Outport
  A_SP_true : Outport  Port=2
  wires:
  P/1 -> [P]
  NSP_true/1 -> [NSP_true]
  A_vect_SP/1 -> [A_vect_SP]
  rho_d_SP/1 -> [rho_d_SP]
  rho_s_SP/1 -> [rho_s_SP]
  S_B/1 -> [S_B]
  Product/1 -> Reshape/1
  [P] -> Gain/1
  Gain/1 -> Product/1
  [S_B] -> Dot Product/2
  [NSP_true] -> Dot Product/1
  Constant/1 -> Add/1
  [rho_s_SP] -> Add/2
  Add/1 -> Product1/1
  [S_B] -> Product1/2
  [rho_s_SP] -> Gain1/1
  [NSP_true] -> Dot Product1/1
  [S_B] -> Dot Product1/2
  Dot Product1/1 -> Product2/2
  Gain1/1 -> Product2/1
  Product2/1 -> Add1/1
  [rho_d_SP] -> Gain2/1
  Gain2/1 -> Add1/2
  [NSP_true] -> Transpose/1
  Add1/1 -> Product3/1
  Product1/1 -> Add2/1
  Product3/1 -> Add2/2
  Transpose/1 -> Product3/2
  Add2/1 -> Product/3
  Reshape/1 -> [F_SP]
  [F_SP] -> F_SP/1
  Dot Product/1 -> Product4/2
  [A_vect_SP] -> Product4/1
  Product4/1 -> [A_SP_true]
  [A_SP_true] -> A_SP_true/1
  [A_SP_true] -> Product/2

== system pointing_group24/Desturbances/External Torques/Solar radiation/Pressure ==
  Constant6 : Constant  Value=1358
  Constant7 : Constant  Value=c
  Product8 : Product
  Reciprocal : Product  Inputs=/
  P : Outport
  wires:
  Constant6/1 -> Product8/1
  Reciprocal/1 -> Product8/2
  Product8/1 -> P/1
  Constant7/1 -> Reciprocal/1

== system pointing_group24/Desturbances/External Torques/Solar radiation/SP center arm ==
  MB : Inport
  SP : Inport  Port=2
  Demux : Demux
  Demux1 : Demux
  Terminator{1..5} (5 alike) : Terminator
  r_SPx : Subsystem
  r_SPy : Subsystem
  r_SP1 : Outport
  r_SP2 : Outport  Port=2
  r_SP3 : Outport  Port=3
  r_SP4 : Outport  Port=4
  wires:
  [a_MB] -> r_SPx/2(a_MB)
  Demux/1 -> Terminator5/1
  SP/1 -> Demux/1
  Demux1/2 -> [a_MB]
  Demux1/3 -> [b_MB]
  Demux1/1 -> Terminator2/1
  Demux1/4 -> Terminator1/1
  MB/1 -> Demux1/1
  Demux/4 -> Terminator3/1
  Demux/2 -> Terminator4/1
  r_SPx/2(r_SP2) -> r_SP2/1
  Demux/3 -> [b_SP]
  [b_SP] -> r_SPx/1(b_SP)
  r_SPx/1(r_SP1) -> r_SP1/1
  r_SPy/1(r_SP1) -> r_SP3/1
  [b_SP] -> r_SPy/1(b_SP)
  r_SPy/2(r_SP2) -> r_SP4/1
  [b_MB] -> r_SPy/2(b_MB)

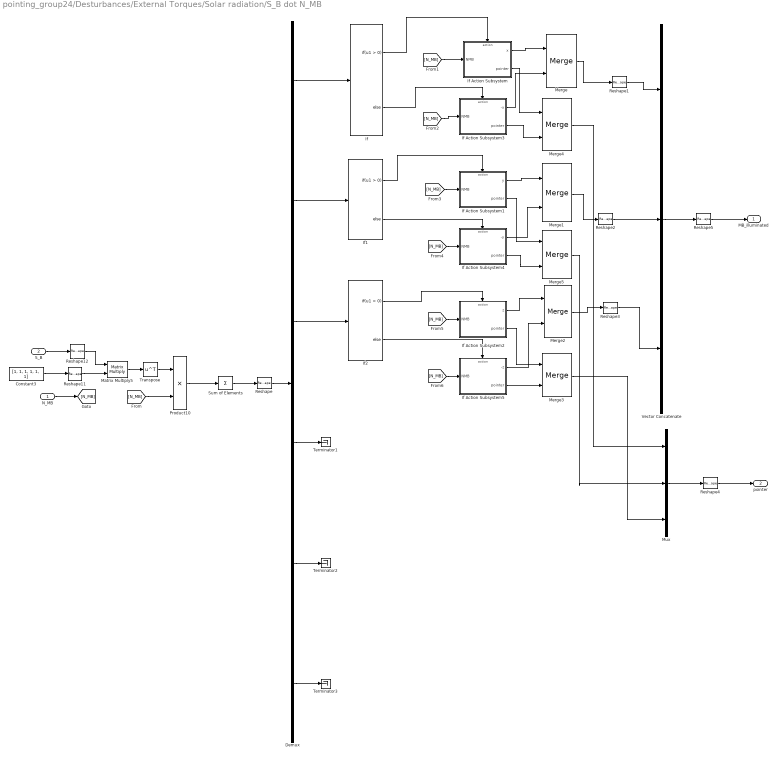
== system pointing_group24/Desturbances/External Torques/Solar radiation/S_B dot N_MB ==
  N_MB : Inport
  S_B : Inport  Port=2
  Constant3 : Constant  Value=[1, 1, 1, 1, 1, 1]  VectorParams1D=off
  Demux : Demux  Outputs=6
  If : If
  If Action Subsystem : Subsystem  TreatAsAtomicUnit=on
  If Action Subsystem1 : Subsystem  TreatAsAtomicUnit=on
  If Action Subsystem2 : Subsystem  TreatAsAtomicUnit=on
  If Action Subsystem3 : Subsystem  TreatAsAtomicUnit=on
  If Action Subsystem4 : Subsystem  TreatAsAtomicUnit=on
  If Action Subsystem5 : Subsystem  TreatAsAtomicUnit=on
  If1 : If
  If2 : If
  Matrix Multiply5 : Product  Multiplication=Matrix(*)
  Merge{,1..5} (6 alike) : Merge
  Mux : Mux  Inputs=3
  Product10 : Product
  Reshape{,1..4,12} (6 alike) : Reshape  OutputDimensionality=Column vector (2-D)
  Reshape11 : Reshape  OutputDimensionality=Row vector (2-D)
  Reshape5 : Reshape  OutputDimensionality=Customize  OutputDimensions=[3,3]
  Sum of Elements : Sum  Inputs=+  CollapseMode=Specified dimension  CollapseDim=2
  Terminator1 : Terminator
  Terminator2 : Terminator
  Terminator3 : Terminator
  Transpose : Math  Operator=transpose
  Vector Concatenate : Concatenate  NumInputs=3
  MB_illuminated : Outport
  pointer : Outport  Port=2
  wires:
  Reshape12/1 -> Matrix Multiply5/1
  Matrix Multiply5/1 -> Transpose/1
  Product10/1 -> Sum of Elements/1
  Reshape11/1 -> Matrix Multiply5/2
  Constant3/1 -> Reshape11/1
  S_B/1 -> Reshape12/1
  Sum of Elements/1 -> Reshape/1
  Reshape/1 -> Demux/1
  Demux/1 -> If/1
  If/1 -> If Action Subsystem/Action
  If/2 -> If Action Subsystem3/Action
  N_MB/1 -> [N_MB]
  [N_MB] -> Product10/2
  [N_MB] -> If Action Subsystem/1(NMB)
  Demux/4 -> Terminator1/1
  Demux/5 -> Terminator2/1
  Demux/6 -> Terminator3/1
  Demux/2 -> If1/1
  If1/1 -> If Action Subsystem1/Action
  [N_MB] -> If Action Subsystem3/1(NMB)
  [N_MB] -> If Action Subsystem1/1(NMB)
  If1/2 -> If Action Subsystem4/Action
  [N_MB] -> If Action Subsystem4/1(NMB)
  If Action Subsystem3/1(-x) -> Merge/2
  If Action Subsystem/1(x) -> Merge/1
  If Action Subsystem1/1(y) -> Merge1/1
  If Action Subsystem2/1(z) -> Merge2/1
  If Action Subsystem5/1(-z) -> Merge2/2
  Demux/3 -> If2/1
  If2/1 -> If Action Subsystem2/Action
  If2/2 -> If Action Subsystem5/Action
  [N_MB] -> If Action Subsystem2/1(NMB)
  [N_MB] -> If Action Subsystem5/1(NMB)
  Merge/1 -> Reshape1/1
  Merge1/1 -> Reshape2/1
  Merge2/1 -> Reshape3/1
  Reshape1/1 -> Vector Concatenate/1
  Reshape2/1 -> Vector Concatenate/2
  Reshape3/1 -> Vector Concatenate/3
  Vector Concatenate/1 -> Reshape5/1
  If Action Subsystem4/1(-y) -> Merge1/2
  If Action Subsystem/2(pointer) -> Merge4/1
  If Action Subsystem3/2(pointer) -> Merge4/2
  If Action Subsystem1/2(pointer) -> Merge5/1
  If Action Subsystem4/2(pointer) -> Merge5/2
  If Action Subsystem2/2(pointer) -> Merge3/1
  If Action Subsystem5/2(pointer) -> Merge3/2
  Merge4/1 -> Mux/1
  Merge5/1 -> Mux/2
  Merge3/1 -> Mux/3
  Mux/1 -> Reshape4/1
  Reshape4/1 -> pointer/1
  Reshape5/1 -> MB_illuminated/1
  Transpose/1 -> Product10/1

== system pointing_group24/Desturbances/External Torques/Solar radiation/S_B dot N_SP ==
  N_SP : Inport
  S_B : Inport  Port=2
  Constant3 : Constant  Value=[1, 1, 1, 1]
  Demux : Demux
  If : If
  If Action Subsystem : Subsystem  TreatAsAtomicUnit=on
  If Action Subsystem1 : Subsystem  TreatAsAtomicUnit=on
  If1 : If
  Matrix Multiply5 : Product  Multiplication=Matrix(*)
  Merge : Merge
  Merge1 : Merge
  Product10 : Product
  Reshape11 : Reshape  OutputDimensionality=Row vector (2-D)
  Reshape12 : Reshape  OutputDimensionality=Column vector (2-D)
  Sum of Elements : Sum  Inputs=+  CollapseMode=Specified dimension  CollapseDim=2
  Terminator{,1..3} (4 alike) : Terminator
  Transpose : Math  Operator=transpose
  SP_illuminated : Outport
  pointer : Outport  Port=2
  wires:
  [N_SP] -> Product10/2
  N_SP/1 -> [N_SP]
  Sum of Elements/1 -> Demux/1
  S_B/1 -> Reshape12/1
  Constant3/1 -> Reshape11/1
  Reshape11/1 -> Matrix Multiply5/2
  Product10/1 -> Sum of Elements/1
  Matrix Multiply5/1 -> Transpose/1
  Reshape12/1 -> Matrix Multiply5/1
  Transpose/1 -> Product10/1
  Demux/1 -> If/1
  If/1 -> If Action Subsystem/Action
  Demux/2 -> If1/1
  [N_SP] -> If Action Subsystem/1(N_SP)
  [N_SP] -> If Action Subsystem1/1(N_SP)
  If1/1 -> If Action Subsystem1/Action
  If1/2 -> Terminator/1
  If/2 -> Terminator1/1
  If Action Subsystem/1(true_NSP) -> Merge/1
  If Action Subsystem1/1(true_NSP) -> Merge/2
  If Action Subsystem/2(pointer) -> Merge1/1
  If Action Subsystem1/2(pointer) -> Merge1/2
  Merge/1 -> SP_illuminated/1
  Merge1/1 -> pointer/1
  Demux/3 -> Terminator2/1
  Demux/4 -> Terminator3/1

== system pointing_group24/Desturbances/External Torques/Solar radiation/Sun position ==
  A_B_N : Inport
  Clock : Clock
  Constant : Constant  Value=2*pi
  Constant1 : Constant  Value=365*24*60*60
  Constant2 : Constant  Value=23.45
  Degrees to Radians : simulink_extras/Transformations/Degrees to Radians
  MatrixMultiply : Product  Multiplication=Matrix(*)
  Mux : Mux  Inputs=3
  Product{,1..3} (4 alike) : Product
  Reciprocal : Product  Inputs=1
  Reshape : Reshape  OutputDimensionality=Column vector (2-D)
  Sin : Trigonometry  Operator=cos
  Sin1 : Trigonometry
  Sin2 : Trigonometry  Operator=cos
  Sin3 : Trigonometry
  S_B : Outport
  wires:
  Product3/1 -> Mux/3
  Degrees to Radians/1 -> Sin3/1, Sin2/1
  Constant1/1 -> Reciprocal/1
  Sin2/1 -> Product2/2
  Product/1 -> Product1/1  "n"
  Constant2/1 -> Degrees to Radians/1
  Product1/1 -> Sin/1, Sin1/1  "n*t"
  Product2/1 -> Mux/2
  Sin3/1 -> Product3/2
  Clock/1 -> Product1/2
  Sin1/1 -> Product3/1, Product2/1
  Constant/1 -> Product/1
  Sin/1 -> Mux/1
  Reciprocal/1 -> Product/2
  Mux/1 -> Reshape/1
  A_B_N/1 -> MatrixMultiply/1
  MatrixMultiply/1 -> S_B/1
  Reshape/1 -> MatrixMultiply/2

== system pointing_group24/Desturbances/External Torques/Solar radiation/Torque arm MB ==
  note: creo il vettore somma che ha per colonna i raggi vettori che collegano il CM del MB con i centri illuminati delle facce nel caso che il sole sia nelle 4 posizioni.
  MB : Inport
  A_vect : Inport  Port=2
  S_B : Inport  Port=3
  pointer : Inport  Port=4
  Demux : Demux  Outputs=3
  Reshape : Reshape  OutputDimensionality=Customize  OutputDimensions=[3,3]
  Transpose : Math  Operator=transpose
  Vector Concatenate : Concatenate  NumInputs=3
  creazione raggi vettore tra CM MB e centro facce illuminate della faccia che ha come normale l'asse i : Subsystem
  creazione raggi vettore tra CM MB e centro facce illuminate della faccia che ha come normale l'asse j : Subsystem
  creazione raggi vettore tra CM MB e centro facce illuminate della faccia che ha come normale l'asse k : Subsystem
  dist : Outport
  wires:
  pointer/1 -> Demux/1
  [x] -> creazione raggi vettore tra CM MB e centro facce illuminate della faccia che ha come normale l'asse i/4(pointer)
  [A_vect] -> creazione raggi vettore tra CM MB e centro facce illuminate della faccia che ha come normale l'asse i/3(A_vect)
  [MB] -> creazione raggi vettore tra CM MB e centro facce illuminate della faccia che ha come normale l'asse k/2(MB)
  [y] -> creazione raggi vettore tra CM MB e centro facce illuminate della faccia che ha come normale l'asse j/4(pointer)
  S_B/1 -> [S_B]
  [A_vect] -> creazione raggi vettore tra CM MB e centro facce illuminate della faccia che ha come normale l'asse k/3(A_vect)
  [MB] -> creazione raggi vettore tra CM MB e centro facce illuminate della faccia che ha come normale l'asse j/2(MB)
  A_vect/1 -> [A_vect]
  MB/1 -> [MB]
  [MB] -> creazione raggi vettore tra CM MB e centro facce illuminate della faccia che ha come normale l'asse i/2(MB)
  Reshape/1 -> Transpose/1
  Transpose/1 -> dist/1
  [S_B] -> creazione raggi vettore tra CM MB e centro facce illuminate della faccia che ha come normale l'asse k/1(S_B)
  Demux/1 -> [x]
  Demux/3 -> [z]
  [S_B] -> creazione raggi vettore tra CM MB e centro facce illuminate della faccia che ha come normale l'asse j/1(S_B)
  [z] -> creazione raggi vettore tra CM MB e centro facce illuminate della faccia che ha come normale l'asse k/4(pointer)
  Vector Concatenate/1 -> Reshape/1  "vectors x, y, z"
  [A_vect] -> creazione raggi vettore tra CM MB e centro facce illuminate della faccia che ha come normale l'asse j/3(A_vect)
  [S_B] -> creazione raggi vettore tra CM MB e centro facce illuminate della faccia che ha come normale l'asse i/1(S_B)
  Demux/2 -> [y]
  creazione raggi vettore tra CM MB e centro facce illuminate della faccia che ha come normale l'asse k/1(Out1) -> Vector Concatenate/3
  creazione raggi vettore tra CM MB e centro facce illuminate della faccia che ha come normale l'asse j/1(Out1) -> Vector Concatenate/2
  creazione raggi vettore tra CM MB e centro facce illuminate della faccia che ha come normale l'asse i/1(Out1) -> Vector Concatenate/1

== system pointing_group24/Desturbances/External Torques/Solar radiation/Torque arm SP ==
  SP : Inport
  A_vect_SP : Inport  Port=2
  S_B : Inport  Port=3
  pointer_SP : Inport  Port=4
  r_SP1 : Inport  Port=5
  r_SP2 : Inport  Port=6
  r_SP3 : Inport  Port=7
  r_SP4 : Inport  Port=8
  Add{,1..3} (4 alike) : Sum
  Reshape : Reshape  OutputDimensionality=Customize  OutputDimensions=[4,3]
  Vector Concatenate : Concatenate  NumInputs=4
  creazione raggi vettore tra CM SP e centro di pressione della faccia illuminata : Subsystem
  distance : Outport
  wires:
  Reshape/1 -> distance/1
  SP/1 -> [SP]
  A_vect_SP/1 -> [A_vect_SP]
  S_B/1 -> [S_B]
  pointer_SP/1 -> [pointer_SP]
  r_SP1/1 -> [r_SP1]
  r_SP2/1 -> [r_SP2]
  [S_B] -> creazione raggi vettore tra CM SP e centro di pressione della faccia illuminata/1(S_B)
  [SP] -> creazione raggi vettore tra CM SP e centro di pressione della faccia illuminata/2(SP)
  [A_vect_SP] -> creazione raggi vettore tra CM SP e centro di pressione della faccia illuminata/3(A_vect)
  [pointer_SP] -> creazione raggi vettore tra CM SP e centro di pressione della faccia illuminata/4(pointer)
  creazione raggi vettore tra CM SP e centro di pressione della faccia illuminata/1(distance_x) -> [distance_x]
  Vector Concatenate/1 -> Reshape/1
  Add/1 -> Vector Concatenate/1
  [distance_x] -> Add/1
  [r_SP1] -> Add/2
  [r_SP2] -> Add1/2
  [distance_x] -> Add1/1
  Add1/1 -> Vector Concatenate/2
  r_SP3/1 -> [r_SP3]
  r_SP4/1 -> [r_SP4]
  Add2/1 -> Vector Concatenate/3
  [distance_y] -> Add2/1
  [r_SP3] -> Add2/2
  [r_SP4] -> Add3/2
  [distance_y] -> Add3/1
  Add3/1 -> Vector Concatenate/4
  creazione raggi vettore tra CM SP e centro di pressione della faccia illuminata/2(distance_y) -> [distance_y]
